simulink model "mfordmodel_v1"  (R2023a)
settings: Solver=ode45  StartTime=0.0  StopTime=10.0  RelTol=1e-3  EnableMultiTasking=on
undefined symbols (not defined in the file): ABV_RATIO_SW, AC_OFF_DLY, ACLOD, AUTO_TRNS_SW, BRAKE_DNDT_X, BZZRPM, BZZRPM_ALT, BZZTM, BZZTM_ALT, CMD_LITOFF, CMD_STABLE, CO_ST_ECT__A, COOL_BASE, DAS_BKDLY_A, DAS_CNT, DAS_CTDLY, DAS_LC_SW__A, DASCLP_5INH, DASCTL, DASMHYST, DASMPH, DEBYCP, DES_BASE, DPNEU_MUL, DSDRPM_DN_TC, DSDRPM_OFF, DSDRPM_UP_TC, EDF_DELAY, EDFHP, ETC_CL_TP, ETC_HP, GR_CM_CREEP, HCAM_ACT_CLP, HEDFHP, HEDFRPM, HICAM_PS, IAC_CAL_SW, IAC_ER_TM1, IAC_ER_TM2, IAC_ER_TM4, IAC_HI_LIM__A, IAC_ISFL_OBD, IAC_KAM_SW, IAC_LO_LIM__A, IAC_MON_TM, IAC_OT_REQ, IAC_RUN_TM, IAC_TP_OBD, IAC_TR_DAS, IAC_TST_DC, ID_DAS__A, ID_NOVS__A, IDVS_CH__A, IDVS_SL__A, IPSI_SW, IPSIDLY, IS_DRBASE__A, IS_DRBASE_A__A, IS_NUBASE__A, IS_NUBASE_A__A ... (+35)
libraries: simulink x2
(part 2 of 12)

== system mfordmodel_v1/iac_v04_001_001/activate_desired_rpm/base_rpm_and_select_logic ==
  note: Note: Be sure to enable C bit-like
      | operations for this chart during test.
  trig_base_rpm_and_select_logic : Inport
  iac_inf_amb : Inport  Port=2
  is_tot_rpm : Inport  Port=3
  is_xtend_rpm : Inport  Port=4
  is_ps_rpm : Inport  Port=5
  is_ac_rpm : Inport  Port=6
  is_alt_rpm : Inport  Port=7
  is_tsl_rpm : Inport  Port=8
  is_hedf_rpm : Inport  Port=9
  er_rpm : Inport  Port=10
  hicam : Inport  Port=11
  dndsup : Inport  Port=12
  alt_cal_flg : Inport  Port=13
  cool_flg : Inport  Port=14
  runup_flg : Inport  Port=15
  iac_dlt_time : Inport  Port=16
  er_isc_req : Inport  Port=17
  base_rpm_and_select_logic_ctl : Stateflow chart  TreatAsAtomicUnit=on
  dsdrpm_calc : Subsystem  TreatAsAtomicUnit=on  mask(do_dsdrpm_calc){}
      mask help: TBD
      mask Display:
      | disp('
      | dsdrpm_lst = dsdrpm;           \n
      | dsdrpm = rolav_tc ( dsdrpm, \n
      |  dsdrpm_tmp,      \n
      |  iac_dlt_time,    \n
      | dsdrpm_tc_tmp)\n
      | ')
  htr_core_rpm_calc : Subsystem  TreatAsAtomicUnit=on  mask(do_htr_core_rpm_calc){}
      mask help: TBD
      mask Display:
      | disp('
      | IF ( ml_heater_core_calc_sw == 1)  THEN        \n
      | is_heater_core_rpm_tmp =               \n
      | fox( FN_NUBASE_IA, iac_inf_amb)\n
      | ELSE IF (ml_heater_core_calc_sw == 2) THEN   \n
      | is_heater_core_rpm_tmp =                \n
      | fox( FN_DRBASE_IA, iac_inf_amb)\n
      | ENDIF                                                          ')
  dsdrpm : Outport
  dsdrpm_lst : Outport  Port=2
  is_source : Outport  Port=3
  wires:
  dsdrpm_calc/2(dsdrpm_lst) -> dsdrpm_lst/1, [dsdrpm_lst]
  [dsdrpm_lst] -> base_rpm_and_select_logic_ctl/14(dsdrpm_lst)
  [do_dsdrpm_calc] -> dsdrpm_calc/Trigger
  iac_dlt_time/1 -> dsdrpm_calc/3(iac_dlt_time)
  base_rpm_and_select_logic_ctl/2(dsdrpm_tmp) -> dsdrpm_calc/1(dsdrpm_tmp)  "dsdrpm_tmp"
  base_rpm_and_select_logic_ctl/3(dsdrpm_tc_tmp) -> dsdrpm_calc/2(dsdrpm_tc_tmp)  "dsdrpm_tc_tmp"
  runup_flg/1 -> base_rpm_and_select_logic_ctl/13(runup_flg)
  cool_flg/1 -> base_rpm_and_select_logic_ctl/12(cool_flg)
  alt_cal_flg/1 -> base_rpm_and_select_logic_ctl/11(alt_cal_flg)
  dndsup/1 -> base_rpm_and_select_logic_ctl/10(dndsup)
  hicam/1 -> base_rpm_and_select_logic_ctl/9(hicam)
  er_rpm/1 -> base_rpm_and_select_logic_ctl/8(er_rpm)
  is_hedf_rpm/1 -> base_rpm_and_select_logic_ctl/7(is_hedf_rpm)
  is_tsl_rpm/1 -> base_rpm_and_select_logic_ctl/6(is_tsl_rpm)
  is_alt_rpm/1 -> base_rpm_and_select_logic_ctl/5(is_alt_rpm)
  is_ac_rpm/1 -> base_rpm_and_select_logic_ctl/4(is_ac_rpm)
  is_ps_rpm/1 -> base_rpm_and_select_logic_ctl/3(is_ps_rpm)
  is_xtend_rpm/1 -> base_rpm_and_select_logic_ctl/2(is_xtend_rpm)
  is_tot_rpm/1 -> base_rpm_and_select_logic_ctl/1(is_tot_rpm)
  htr_core_rpm_calc/1(is_heater_core_rpm_tmp) -> base_rpm_and_select_logic_ctl/16(is_heater_core_rpm_tmp)
  base_rpm_and_select_logic_ctl/4(ml_htr_core_calc_sw) -> htr_core_rpm_calc/1(ml_heater_core_calc_sw)  "ml_heater_core_calc_sw"
  iac_inf_amb/1 -> htr_core_rpm_calc/2(iac_inf_amb)
  base_rpm_and_select_logic_ctl/6(do_htr_core_rpm_calc()) -> htr_core_rpm_calc/Trigger  "do_htr_core_rpm_calc"
  base_rpm_and_select_logic_ctl/1(is_source) -> is_source/1  "is_source"
  base_rpm_and_select_logic_ctl/5(do_dsdrpm_calc()) -> [do_dsdrpm_calc]  "do_dsdrpm_calc"
  trig_base_rpm_and_select_logic/1 -> base_rpm_and_select_logic_ctl/Trigger
  er_isc_req/1 -> base_rpm_and_select_logic_ctl/15(er_isc_req)
  dsdrpm_calc/1(dsdrpm) -> dsdrpm/1

== system mfordmodel_v1/iac_v04_001_001/activate_desired_rpm/hicam_rpm_request ==
  note: Note: Be sure to enable C bit-like
      | operations for this chart during test.
  trig_hicam_rpm_request : Inport
  act : Inport  Port=2
  ect : Inport  Port=3
  acstrt : Inport  Port=4
  tcstrt : Inport  Port=5
  atmr1 : Inport  Port=6
  apt : Inport  Port=7
  crkflg : Inport  Port=8
  ndsflg : Inport  Port=9
  dndsup : Inport  Port=10
  ext_cmd : Inport  Port=11
  alt_cal_flg : Inport  Port=12
  iac_dlt_time : Inport  Port=13
  runup_flg : Inport  Port=14
  fox_calcs : Subsystem  TreatAsAtomicUnit=on  mask(fox_calcs){}
      mask help: TBD
      mask Display:
      | disp('\n
      | ml_fn825b = FN825b(act)               \n
      | ml_fn826b = FN826B(act)               \n
      | ml_fn803a = FN803A(acstrt            \n
      | ml_fn826a = FN826A(tcstrt)            \n
      | ml_fn825a = FN825A(ect)               \n
      | ml_fn825a_alt = FN825A_ALT(ect)\n\n
      | ml_isadd_min = MIN( ml_fn825b,   \n
      | HCAM_ACT_CLP) ')
  hicam_calc : Subsystem  TreatAsAtomicUnit=on  mask(hicam_calc){}
      mask help: TBD
      mask Display:
      | disp('\n
      | IF (ml_isadd_sw == 1) THEN           \n
      |   isadd_ext__A = IS_CMD_ADD \n
      | ELSE IF (ml_isadd_sw == 2) THEN \n
      |   isadd_ext__A = ml_isadd_ext \n
      | ELSE IF (ml_isadd_sw == 3) THEN \n
      |   isadd_ext__A = 0.0                  \n
      | ENDIF                                             \n\n
      | hicam =   isadd_act_tmp                \n
      |                + isadd_ect_tmp     \n
      |                + isadd_st_ect_tmp \n
      |                + isadd_st_act_tmp \n
      |                + isadd_buzz_tmp   \n
      |                + isadd_ext__A        ')
  hicam_rpm_request_ctl : Stateflow chart  TreatAsAtomicUnit=on
  isadd_ramp : Subsystem  TreatAsAtomicUnit=on  mask(isadd_ramp){}
      mask help: If the CAT is cold and the engine is running then ramp the CAT mid rpm adder up. If the CAT is warm (out of deadban) then ramp the rpm adder towards zero because no rpm adder is needed.
      mask Display:
      | disp('\n
      | IF (ml_ramp_sw == 1) THEN               \n
      |  ramp ml_isadd_ext towards          \n
      |  IS_CMD_ADD  with TC = 60 sec. \n
      | ELSE (ml_ramp_sw == 2) THEN         \n
      |   ramp ml_isadd_ext towards         \n
      |   0.0  with TC = 30 sec.                 \n
      | ENDIF                                                 \n
      | ')
  hicam : Outport
  ctptfg : Outport  Port=2
  ptctfg : Outport  Port=3
  wires:
  ext_cmd/1 -> hicam_rpm_request_ctl/7(ext_cmd)
  dndsup/1 -> hicam_rpm_request_ctl/6(dndsup)
  hicam_rpm_request_ctl/9(ptctfg) -> ptctfg/1  "ptctfg"
  hicam_rpm_request_ctl/8(ctptfg) -> ctptfg/1  "ctptfg"
  ndsflg/1 -> hicam_rpm_request_ctl/5(ndsflg)
  crkflg/1 -> hicam_rpm_request_ctl/4(crkflg)
  apt/1 -> hicam_rpm_request_ctl/3(apt)
  atmr1/1 -> hicam_rpm_request_ctl/2(atmr1)
  alt_cal_flg/1 -> hicam_rpm_request_ctl/1(alt_cal_flg)
  fox_calcs/6(ml_fn825a_alt) -> hicam_rpm_request_ctl/10(ml_fn825a_alt)
  fox_calcs/5(ml_fn825a) -> hicam_rpm_request_ctl/11(ml_fn825a)
  fox_calcs/4(ml_fn826b) -> hicam_rpm_request_ctl/12(ml_fn826b)
  fox_calcs/3(ml_fn826a) -> hicam_rpm_request_ctl/13(ml_fn826a)
  fox_calcs/2(ml_fn803a) -> hicam_rpm_request_ctl/14(ml_fn803a)
  fox_calcs/1(ml_fn825b) -> hicam_rpm_request_ctl/15(ml_fn825b)
  hicam_rpm_request_ctl/10(do_hicam_calc()) -> [do_hicam_calc]  "do_hicam_calc"
  trig_hicam_rpm_request/1 -> hicam_rpm_request_ctl/Trigger
  hicam_rpm_request_ctl/12(do_fox_calcs()) -> fox_calcs/Trigger  "do_fox_calcs"
  hicam_rpm_request_ctl/5(isadd_buzz_tmp) -> hicam_calc/5(isadd_buzz_tmp)  "isadd_buzz_tmp"
  hicam_rpm_request_ctl/4(isadd_st_act_tmp) -> hicam_calc/4(isadd_st_act_tmp)  "isadd_st_act_tmp"
  hicam_rpm_request_ctl/3(isadd_st_ect_tmp) -> hicam_calc/3(isadd_st_ect_tmp)  "isadd_st_ect_tmp"
  hicam_rpm_request_ctl/2(isadd_ect_tmp) -> hicam_calc/2(isadd_ect_tmp)  "isadd_ect_tmp"
  hicam_rpm_request_ctl/1(isadd_act_tmp) -> hicam_calc/1(isadd_act_tmp)  "isadd_act_tmp"
  [do_hicam_calc] -> hicam_calc/Trigger
  fox_calcs/7(ml_isadd_min) -> hicam_rpm_request_ctl/9(ml_isadd_min)
  hicam_rpm_request_ctl/6(ml_isadd_sw) -> hicam_calc/6(ml_isadd_sw)  "ml_isadd_sw"
  hicam_rpm_request_ctl/11(do_isadd_ramp()) -> [do_isadd_ramp]  "do_isadd_ramp"
  isadd_ramp/1(ml_isadd_ext) -> hicam_calc/7(ml_isadd_ext)
  hicam_rpm_request_ctl/7(ml_ramp_sw) -> [ml_ramp_sw]  "ml_ramp_sw"
  tcstrt/1 -> fox_calcs/3(tcstrt)
  act/1 -> fox_calcs/1(act)
  runup_flg/1 -> hicam_rpm_request_ctl/8(runup_flg)
  [do_isadd_ramp] -> isadd_ramp/Trigger
  [isadd_ext__A] -> isadd_ramp/2(isadd_ext__A)
  [ml_ramp_sw] -> isadd_ramp/1(ml_ramp_sw)
  iac_dlt_time/1 -> isadd_ramp/3(iac_dlt_time)
  ect/1 -> fox_calcs/4(ect)
  acstrt/1 -> fox_calcs/2(acstrt)
  hicam_calc/1(hicam) -> hicam/1
  hicam_calc/2(isadd_ext__A) -> [isadd_ext__A]

== system mfordmodel_v1/iac_v04_001_001/activate_desired_rpm/inf_amb_calc ==
  ml_inf_amb_sw : Inport
  infamb_kam : Inport  Port=2
  iac_dlt_time : Inport  Port=3
  do_inf_amb_calc : TriggerPort  TriggerType=function-call  VariantControl=(inherit)
  Constant : Constant  Value=254.0
  Multiport Switch : MultiPortSwitch  Inputs=2
  ROLAV_TC_DT_in : Subsystem  mask(Rolling Average - Time Constant){TAU=16}
      mask prompts: TAU "Time Constant"
      mask help: Rolling Average - Time Constant. This filter block is the first order approximation using a time constant. Inputs include the time constant (entered through this dialogue), old_ave which is the previous average value, new_value which is the new filter to filter toward, and the delta_time which is elapsed time over which to perform the filter equation.
      mask init:
      | if isletter(TAU(1))
      |   tc = evalin('base',TAU);
      |   name = TAU;
      | else
      |   tc = str2num(TAU);
      |   name = 'TC';
      | end;
      mask Display: fprintf('%s = %.4f',name,tc);
  Unit Delay : UnitDelay  SampleTime=-1
  iac_inf_amb : Outport
  wires:
  Multiport Switch/1 -> iac_inf_amb/1, Unit Delay/1  "iac_inf_amb"
  ml_inf_amb_sw/1 -> Multiport Switch/1
  infamb_kam/1 -> Multiport Switch/2
  ROLAV_TC_DT_in/1(new_ave) -> Multiport Switch/3  "iac_inf_amb"
  iac_dlt_time/1 -> ROLAV_TC_DT_in/3(delta_time)
  Constant/1 -> ROLAV_TC_DT_in/1(new_value)
  Unit Delay/1 -> ROLAV_TC_DT_in/2(old_ave)

== system mfordmodel_v1/iac_v04_001_001/activate_desired_rpm/rpm_adders_fans_and_pw_steer ==
  trig_rpm_adders_fans_pw_steer : Inport
  hsf_flg : Inport  Port=2
  powsfg : Inport  Port=3
  rpm_adders_fans_pw_steer_ctl : Stateflow chart  TreatAsAtomicUnit=on
  is_hedf_rpm : Outport
  is_ps_rpm : Outport  Port=2
  wires:
  powsfg/1 -> rpm_adders_fans_pw_steer_ctl/2(powsfg)
  hsf_flg/1 -> rpm_adders_fans_pw_steer_ctl/1(hsf_flg)
  rpm_adders_fans_pw_steer_ctl/1(is_hedf_rpm) -> is_hedf_rpm/1  "is_hedf_rpm"
  rpm_adders_fans_pw_steer_ctl/2(is_ps_rpm) -> is_ps_rpm/1  "is_ps_rpm"
  trig_rpm_adders_fans_pw_steer/1 -> rpm_adders_fans_pw_steer_ctl/Trigger

== system mfordmodel_v1/iac_v04_001_001/activate_desired_rpm/rpm_calcs ==
  nobart : Inport
  stb_lold_tmr : Inport  Port=2
  tot : Inport  Port=3
  iac_inf_amb : Inport  Port=4
  ml_tsl_sw : Inport  Port=5
  ml_ac_sw : Inport  Port=6
  ml_xtend_sw : Inport  Port=7
  ml_tot_sw : Inport  Port=8
  do_rpm_calcs : TriggerPort  TriggerType=function-call  VariantControl=(inherit)
  "  4" : Subsystem  mask(Constant){constant=COAST_FRAC}
      mask help: Constant Block. Will dispaly constant name and value on the icon of the block
      mask init:
      | if isletter(constant(1))
      |   const = evalin('base',constant);
      |   name = constant;
      | else
      |   const = str2num(constant);
      |   name = 'CONST';
      | end;
      mask Display: fprintf('%s = %.4f',name,const);
  "  5" : Subsystem  mask(Constant){constant=RT_CHAIN}
      mask help: Constant Block. Will dispaly constant name and value on the icon of the block
      mask init:
      | if isletter(constant(1))
      |   const = evalin('base',constant);
      |   name = constant;
      | else
      |   const = str2num(constant);
      |   name = 'CONST';
      | end;
      mask Display: fprintf('%s = %.4f',name,const);
  Constant : Constant  Value=0.0
  Constant1 : Constant  Value=0.0
  Constant2 : Constant  Value=0.0
  Multiport Switch : MultiPortSwitch  Inputs=2
  Multiport Switch1 : MultiPortSwitch
  Multiport Switch2 : MultiPortSwitch  Inputs=2
  Multiport Switch3 : MultiPortSwitch  Inputs=2
  Product : Product  Inputs=3  InputSameDT=on  RndMeth=Zero  SaturateOnIntegerOverflow=on  OutDataTypeStr=Inherit: Same as first input
  lookup_2d : Subsystem  mask(2-D, piece-wise, linear interpolation){CAL_FUNC=FNIAC_AC_N}
      mask prompts: CAL_FUNC "Calibration function name"
      mask help:
      | Performs piece-wise linear interpolation.
      |
      | Output is NOT extrapolated beyond the input range.  If the input value presented to the block lies outside the range specified in the block's parameter, then the value is treated as though it has the value of the nearest value in the range.
      mask init:
      | if isempty(CAL_FUNC) |  isspace(CAL_FUNC)
      |  calfunc.X=[0 5 10];
      |  calfunc.Y=[0 5 10];
      |  min_x=0;
      |  min_y=0;
      |  max_x=10;
      |  max_y=10;
      |  CAL_FUNC='FNxxx';
      | else
      |   calfunc = evalin('base', CAL_FUNC);
      |   min_x = calfunc.X(1);
      |   min_y = calfunc.Y(1);
      |   max_x = calfunc.X(length(calfunc.X));
      |   max_y = calfunc.Y(length(calfunc.Y));
      | end
      mask Help:
      | Enter the name of the calibration function.
      | (e.g. EGM_VA_ECT_MULT)
      mask Display:
      | fprintf('%s',CAL_FUNC);
      | plot(calfunc.X,calfunc.Y,max_x*1.05,max_y*1.05,min_x,min_y);
  lookup_2d1 : Subsystem  mask(2-D, piece-wise, linear interpolation){CAL_FUNC=FNIAC_AC_D}
      mask prompts: CAL_FUNC "Calibration function name"
      mask help:
      | Performs piece-wise linear interpolation.
      |
      | Output is NOT extrapolated beyond the input range.  If the input value presented to the block lies outside the range specified in the block's parameter, then the value is treated as though it has the value of the nearest value in the range.
      mask init: same as mfordmodel_v1/iac_v04_001_001/activate_desired_rpm/rpm_calcs/lookup_2d
      mask Help:
      | Enter the name of the calibration function.
      | (e.g. EGM_VA_ECT_MULT)
      mask Display:
      | fprintf('%s',CAL_FUNC);
      | plot(calfunc.X,calfunc.Y,max_x*1.05,max_y*1.05,min_x,min_y);
  lookup_2d2 : Subsystem  mask(2-D, piece-wise, linear interpolation){CAL_FUNC=FN861R}
      mask prompts: CAL_FUNC "Calibration function name"
      mask help:
      | Performs piece-wise linear interpolation.
      |
      | Output is NOT extrapolated beyond the input range.  If the input value presented to the block lies outside the range specified in the block's parameter, then the value is treated as though it has the value of the nearest value in the range.
      mask init: same as mfordmodel_v1/iac_v04_001_001/activate_desired_rpm/rpm_calcs/lookup_2d
      mask Help:
      | Enter the name of the calibration function.
      | (e.g. EGM_VA_ECT_MULT)
      mask Display:
      | fprintf('%s',CAL_FUNC);
      | plot(calfunc.X,calfunc.Y,max_x*1.05,max_y*1.05,min_x,min_y);
  lookup_2d3 : Subsystem  mask(2-D, piece-wise, linear interpolation){CAL_FUNC=FN861}
      mask prompts: CAL_FUNC "Calibration function name"
      mask help:
      | Performs piece-wise linear interpolation.
      |
      | Output is NOT extrapolated beyond the input range.  If the input value presented to the block lies outside the range specified in the block's parameter, then the value is treated as though it has the value of the nearest value in the range.
      mask init: same as mfordmodel_v1/iac_v04_001_001/activate_desired_rpm/rpm_calcs/lookup_2d
      mask Help:
      | Enter the name of the calibration function.
      | (e.g. EGM_VA_ECT_MULT)
      mask Display:
      | fprintf('%s',CAL_FUNC);
      | plot(calfunc.X,calfunc.Y,max_x*1.05,max_y*1.05,min_x,min_y);
  lookup_2d4 : Subsystem  mask(2-D, piece-wise, linear interpolation){CAL_FUNC=FN880N}
      mask prompts: CAL_FUNC "Calibration function name"
      mask help:
      | Performs piece-wise linear interpolation.
      |
      | Output is NOT extrapolated beyond the input range.  If the input value presented to the block lies outside the range specified in the block's parameter, then the value is treated as though it has the value of the nearest value in the range.
      mask init: same as mfordmodel_v1/iac_v04_001_001/activate_desired_rpm/rpm_calcs/lookup_2d
      mask Help:
      | Enter the name of the calibration function.
      | (e.g. EGM_VA_ECT_MULT)
      mask Display:
      | fprintf('%s',CAL_FUNC);
      | plot(calfunc.X,calfunc.Y,max_x*1.05,max_y*1.05,min_x,min_y);
  is_tsl_rpm : Outport
  is_ac_rpm : Outport  Port=2
  is_tot_rpm : Outport  Port=3
  is_xtend_rpm : Outport  Port=4
  wires:
  "  5"/1(Out) -> Product/2
  Multiport Switch1/1 -> is_ac_rpm/1  "is_ac_rpm"
  Constant1/1 -> Multiport Switch1/4
  lookup_2d/1(Out1) -> Multiport Switch1/2
  lookup_2d1/1(Out1) -> Multiport Switch1/3
  ml_ac_sw/1 -> Multiport Switch1/1
  iac_inf_amb/1 -> lookup_2d/1(In1), lookup_2d1/1(In1)
  "  4"/1(Out) -> Product/3
  nobart/1 -> Product/1
  lookup_2d2/1(Out1) -> Multiport Switch2/2
  lookup_2d3/1(Out1) -> Multiport Switch2/3
  Multiport Switch2/1 -> is_tot_rpm/1  "is_tot_rpm"
  ml_tot_sw/1 -> Multiport Switch2/1
  tot/1 -> lookup_2d2/1(In1), lookup_2d3/1(In1)
  Constant2/1 -> Multiport Switch3/3
  lookup_2d4/1(Out1) -> Multiport Switch3/2
  Multiport Switch3/1 -> is_xtend_rpm/1  "is_xtend_rpm"
  ml_xtend_sw/1 -> Multiport Switch3/1
  stb_lold_tmr/1 -> lookup_2d4/1(In1)
  Product/1 -> Multiport Switch/3
  Constant/1 -> Multiport Switch/2
  Multiport Switch/1 -> is_tsl_rpm/1  "is_tsl_rpm"
  ml_tsl_sw/1 -> Multiport Switch/1

== system mfordmodel_v1/iac_v04_001_001/iac_executive/fault_code_setting ==
  note: NOTE: Enable 'C-like' bit operations
      | when performing UNIT TEST
      | on this chart.
  trig_fault_code_setting : Inport
  abv_percent : Inport  Port=2
  abv_status : Inport  Port=3
  ccm_ena_flg : Inport  Port=4
  iac_dlt_time : Inport  Port=5
  Constant3 : Constant  Value=0.0
  Constant4 : Constant  Value=0
  Constant5 : Constant
  TIMER_DT_in : Subsystem  mask(TIMER){timer_name=iac_er_tmr4, init_value=0, clipped=off, tmin=, tmax=, unit_str=seconds}
      mask prompts: timer_name "Enter Timer Name"; init_value "initial TIMER value (in seconds)"; clipped "Clip timer?"; tmin "Minimum clip"; tmax "Maximum clip"; unit_str "Select timer units"
      mask help: Acts as a timer. Can count up, down, hold, or reset to zero. The required inputs are a timer function call, a reset function call, a reset value, an increment flag, and a decrement flag. Timer initial value, max and min clip values and timer name are selected below.
      mask init:
      | if ( clipped )
      |   if isletter(tmin(1))
      |     timer_min = evalin('base', tmin);
      |     const_min = timer_min;
      |   else
      |     timer_min = tmin;
      |     tmin = 'Min';
      |     const_min = str2num(timer_min);
      |   end
      |   if isletter(tmax(1))
      |     timer_max = evalin('base', tmax);
      |     const_max = timer_max;
      |   else
      |     timer_max = tmax;
      |     tmax = 'Max';
      |     const_max = str2num(timer_max);
      |   end
      | else
      |   timer_min = 0.0;
      |   const_min = 0.0;
      |   tmin = 'Min';
      |   timer_max = inf;
      |   const_max = inf;
      |    tmax = 'Max';
      | end
      | min_text = strcat(tmin,' = ',num2str(timer_min));
      | max_text = strcat(tmax ,' = ' ,num2str(timer_max));
      | if (strcmp(unit_str, 'seconds' ))
      |   unit_mul = 1;
      |   resolution = 0.000001;
      | else
      |   unit_mul = 1000;
      |    resolution = 1;
      | end
      mask Help:
      | <b><font size="+2">Input/Output Ports</font></b><br>
      | <p>
      | <b>Trig_timer:</b><br>
      | Connect a function call input to the 'trig_timer' port.  A function call passed through this port will activate the TIMER tool.  Activation updates the TIMER output.
      | <p>
      | <b>Trig_reset:</b><br>
      | Connect a function call input to the 'trig_reset' port.  A function call passed through this port will activate the TIMER tool.  Activation resets the TIMER output to the value passed to the 'reset_value' port.
      | <p>
      | <b>Reset_value:</b><br>
      | When 'trig_reset' is activated, the TIMER value will be reset to the real value passed to this input.
      | <p>
      | <b>Increment_flag and decrement_flag:</b><br>
      | If 'increment_flag' is 1 and 'decrement_flag' is 0, TIMER counts up.
      | If 'decrement_flag' is 1 and 'increment_flag' is 0, TIMER counts down.
      | If the flags are both 0 or both 1, TIMER holds its current value.
      | <p>
      | <b><font size="+2">Parameter Selection:</font></b>
      | <p>
      | <b>Initial TIMER Value:</b><br>
      | TIMER will begin at specified value.  Enter in seconds.
      mask TypeOptions unit_str: seconds | milliseconds
      mask Display:
      | plot( [0.3 0.45 0.55 0.7], [0.4 0.4 0.6 0.6])
      | plot( [ .475 .435 .415  .4 .4  .415 .435 .475  .525 .565 .585 .6 .6  ...
      | .585 .565 .525 .475], [.9  .885 .865  .825 .775 .735 .715  .7 .7 ...
      | .715 .735 .775 .825  .865 .885 .9 .9] )
      | plot( [.5 .5], [.89 .87])
      | plot( [.5 .5], [.71 .73])
      | plot( [.41 .43], [.8 .8])
      | plot( [.57 .59], [.8 .8])
      | plot( [.5 .5], [.8 .89])
      | plot( [.49 .5 .51], [.88 .89 .88] )
      | plot( [.5 .555], [.8 .825] )
      | plot( [.535 .555 .555], [.825 .825 .815])
      | text(0.35, 0.35, min_text)
      | text(0.6, 0.7,max_text)
      | text( 0.35, .95, timer_name)
  fault_code_setting_ctl : Stateflow chart  TreatAsAtomicUnit=on
  type1_fault_code : Subsystem  mask(fault code){pcode=1504, ms=CCM}
      mask prompts: pcode "Code Number (e.g. 1234)"; ms "System ID"
      mask help: Gereric Fault Code - NOT functional
      mask init:
      | if (pcode == 'xxxx')
      | pcode_num = 0;
      | else
      | pcode_num = str2num(pcode);
      | end
      | mon_select=eval('ms');
      mask TypeOptions ms: CCM | CAT | PURG | SAIR | EGR | EGO | COOL | FCAP | P0456
      mask Display: fprintf('P%s\n%s',pcode,ms);
  p1504 : Outport
  wires:
  type1_fault_code/1(pxxxx) -> p1504/1  "p1504"
  Constant5/1 -> TIMER_DT_in/4(inc flag)
  Constant4/1 -> TIMER_DT_in/5(dec flag)
  Constant3/1 -> TIMER_DT_in/3(reset value)
  iac_dlt_time/1 -> TIMER_DT_in/6(delta time)
  fault_code_setting_ctl/1(trig_incr_tmr4()) -> TIMER_DT_in/1(trig_time)  "trig_incr_tmr4"
  fault_code_setting_ctl/2(trig_rst_tmr4()) -> TIMER_DT_in/2(trig_reset)  "trig_rst_tmr4"
  TIMER_DT_in/1(timer) -> fault_code_setting_ctl/4(iac_er_tmr4)  "iac_er_tmr4"
  trig_fault_code_setting/1 -> fault_code_setting_ctl/Trigger
  fault_code_setting_ctl/3(trig_set_p1504_malf()) -> type1_fault_code/1(trig_malfunction)  "trig_set_p1504_malf"
  fault_code_setting_ctl/4(trig_clear_p1504_malf()) -> type1_fault_code/2(trig_clear_malf)  "trig_clear_p1504_malf"
  ccm_ena_flg/1 -> fault_code_setting_ctl/3(ccm_ena_flg)
  abv_status/1 -> fault_code_setting_ctl/2(abv_status)
  abv_percent/1 -> fault_code_setting_ctl/1(abv_percent)

== system mfordmodel_v1/iac_v04_001_001/iac_executive/iac_dlt_time_calc ==
  do_iac_dlt_time_calc : TriggerPort  TriggerType=function-call  VariantControl=(inherit)
  Digital Clock : DigitalClock  SampleTime=-1
  Sum : Sum  Inputs=+-  InputSameDT=on  SaturateOnIntegerOverflow=on  OutDataTypeStr=Inherit: Same as first input
  Unit Delay : UnitDelay  SampleTime=-1
  iac_dlt_time : Outport  InitialOutput=0
  wires:
  Digital Clock/1 -> Unit Delay/1, Sum/1
  Sum/1 -> iac_dlt_time/1  "iac_dlt_time"
  Unit Delay/1 -> Sum/2

== system mfordmodel_v1/iac_v04_001_001/iac_executive/misc_calcs ==
  trig_misc_calcs : Inport
  dndti : Inport  Port=2
  iac_dlt_time : Inport  Port=3
  subst_req_0 : Inport  Port=4
  tslpip : Inport  Port=5
  runup_flg : Inport  Port=6
  crkflg : Inport  Port=7
  er_isc_hld : Inport  Port=8
  mfmflg : Inport  Port=9
  tfmflg : Inport  Port=10
  eng_stalled : Inport  Port=11
  gr_cm : Inport  Port=12
  apt : Inport  Port=13
  Constant3 : Constant  Value=0.0
  Constant4 : Constant  Value=0
  Constant5 : Constant
  TIMER_DT_in : Subsystem  mask(TIMER){timer_name=gear5tmr, init_value=0, clipped=on, tmin=0, tmax=31.75, unit_str=seconds}
      mask prompts: timer_name "Enter Timer Name"; init_value "initial TIMER value (in seconds)"; clipped "Clip timer?"; tmin "Minimum clip"; tmax "Maximum clip"; unit_str "Select timer units"
      mask help: Acts as a timer. Can count up, down, hold, or reset to zero. The required inputs are a timer function call, a reset function call, a reset value, an increment flag, and a decrement flag. Timer initial value, max and min clip values and timer name are selected below.
      mask init: same as mfordmodel_v1/iac_v04_001_001/iac_executive/fault_code_setting/TIMER_DT_in
      mask Help:
      | <b><font size="+2">Input/Output Ports</font></b><br>
      | <p>
      | <b>Trig_timer:</b><br>
      | Connect a function call input to the 'trig_timer' port.  A function call passed through this port will activate the TIMER tool.  Activation updates the TIMER output.
      | <p>
      | <b>Trig_reset:</b><br>
      | Connect a function call input to the 'trig_reset' port.  A function call passed through this port will activate the TIMER tool.  Activation resets the TIMER output to the value passed to the 'reset_value' port.
      | <p>
      | <b>Reset_value:</b><br>
      | When 'trig_reset' is activated, the TIMER value will be reset to the real value passed to this input.
      | <p>
      | <b>Increment_flag and decrement_flag:</b><br>
      | If 'increment_flag' is 1 and 'decrement_flag' is 0, TIMER counts up.
      | If 'decrement_flag' is 1 and 'increment_flag' is 0, TIMER counts down.
      | If the flags are both 0 or both 1, TIMER holds its current value.
      | <p>
      | <b><font size="+2">Parameter Selection:</font></b>
      | <p>
      | <b>Initial TIMER Value:</b><br>
      | TIMER will begin at specified value.  Enter in seconds.
      mask TypeOptions unit_str: seconds | milliseconds
      mask Display:
      | plot( [0.3 0.45 0.55 0.7], [0.4 0.4 0.6 0.6])
      | plot( [ .475 .435 .415  .4 .4  .415 .435 .475  .525 .565 .585 .6 .6  ...
      | .585 .565 .525 .475], [.9  .885 .865  .825 .775 .735 .715  .7 .7 ...
      | .715 .735 .775 .825  .865 .885 .9 .9] )
      | plot( [.5 .5], [.89 .87])
      | plot( [.5 .5], [.71 .73])
      | plot( [.41 .43], [.8 .8])
      | plot( [.57 .59], [.8 .8])
      | plot( [.5 .5], [.8 .89])
      | plot( [.49 .5 .51], [.88 .89 .88] )
      | plot( [.5 .555], [.8 .825] )
      | plot( [.535 .555 .555], [.825 .825 .815])
      | text(0.35, 0.35, min_text)
      | text(0.6, 0.7,max_text)
      | text( 0.35, .95, timer_name)
  dndt_calc : Subsystem  TreatAsAtomicUnit=on  mask(dndt_calc){}
      mask help: Filter the rate of change of RPM for use in DASPOT calculations.
      mask Display:
      | disp('\n
      | IF (ml_dndt_sw == 1) THEN          \n
      | dndt_das = 0.0                       \n
      | ELSE IF (ml_dndt_sw == 2) THEN\n
      | dndt_das =  rolav( dndt_das,  \n
      | dndti, iac_dlt_time,\n
      | TCNDT_DAS)          \n
      | ENDIF                                            ')
  misc_calcs_ctl : Stateflow chart  TreatAsAtomicUnit=on
  osc_response_logic_ctl : Stateflow chart  TreatAsAtomicUnit=on
  osc_response_triggered : Subsystem  TreatAsAtomicUnit=on  mask(substitute){resp=22, channel=0}
      mask prompts: resp "Enter Response Code in HEX"; channel "Select OSC channel"
      mask help:
      | This block will perform Output State Control Response, for now it is stub block.
      | Enter the response code and OSC channel number below.
      mask TypeOptions channel: 0 | 1 | 2 | 3 | 4 | 5 | 6 | 7 | 8 | 9 | 10 | 11 | 12 | 15 | 16 | 17 | 18 | 19 | 20 | 21 | 22 | 23 | 24 | 25 | 26 | 27 | 28 | 29 | 30 | 31 | 32 | 33 | 34 | 35 | 36 | 37 | 38 | 39 | 40 | 41 | 42 | 43 | 44 | 45 | 46 | 47 | 48 | 49 | 50
      mask Display: fprintf('\nChannel # = %s\nResponse Code = 0x%s\n',channel,resp);
  gear5tmr : Outport
  gear5th : Outport  Port=2
  dndt_das : Outport  Port=3
  wires:
  apt/1 -> misc_calcs_ctl/3(apt)
  gr_cm/1 -> misc_calcs_ctl/2(gr_cm)
  eng_stalled/1 -> misc_calcs_ctl/1(eng_stalled)
  tslpip/1 -> osc_response_logic_ctl/7(tslpip)
  tfmflg/1 -> osc_response_logic_ctl/6(tfmflg)
  subst_req_0/1 -> osc_response_logic_ctl/5(subst_req_0)
  mfmflg/1 -> osc_response_logic_ctl/4(mfmflg)
  er_isc_hld/1 -> osc_response_logic_ctl/3(er_isc_hld)
  crkflg/1 -> osc_response_logic_ctl/2(crkflg)
  runup_flg/1 -> osc_response_logic_ctl/1(runup_flg)
  misc_calcs_ctl/6(trig_osc_response_logic()) -> osc_response_logic_ctl/Trigger  "trig_osc_response_logic"
  osc_response_logic_ctl/1(do_osc_response()) -> osc_response_triggered/Trigger  "do_osc_responnse"
  dndti/1 -> dndt_calc/2(dndti)
  [ml_dndt_sw] -> dndt_calc/1(ml_dndt_sw)
  misc_calcs_ctl/2(ml_dndt_sw) -> [ml_dndt_sw]  "ml_dndt_sw"
  dndt_calc/1(dndt_das) -> dndt_das/1
  iac_dlt_time/1 -> dndt_calc/3(iac_dlt_time), TIMER_DT_in/6(delta time)
  misc_calcs_ctl/5(do_dndt_calc()) -> dndt_calc/Trigger  "do_dndt_calc"
  Constant3/1 -> TIMER_DT_in/3(reset value)
  Constant4/1 -> TIMER_DT_in/5(dec flag)
  Constant5/1 -> TIMER_DT_in/4(inc flag)
  misc_calcs_ctl/1(gear5th) -> gear5th/1  "gear5th"
  TIMER_DT_in/1(timer) -> gear5tmr/1  "gear5tmr"
  trig_misc_calcs/1 -> misc_calcs_ctl/Trigger
  misc_calcs_ctl/4(trig_rst_gear5tmr()) -> TIMER_DT_in/2(trig_reset)  "trig_rst_gear5tmr"
  misc_calcs_ctl/3(trig_incr_gear5tmr()) -> TIMER_DT_in/1(trig_time)  "trig_incr_gear5tmr"

== system mfordmodel_v1/iac_v04_001_001/iac_executive/mode_control ==
  trig_external_override_mode : Inport
  trig_crank_mode : Inport  Port=2
  do_failure_mode : Inport  Port=3
  osm_eo_off : Inport  Port=4
  osm_eo_on : Inport  Port=5
  osc_ena_0 : Inport  Port=6
  osc_state : Inport  Port=7
  tcstrt : Inport  Port=8
  tslpip : Inport  Port=9
  abv_flowrate_in : Inport  Port=10
  ratch : Inport  Port=11
  abv_ratio_in : Inport  Port=12
  Mux3 : Mux  Inputs=3
  Mux4 : Mux  Inputs=3
  Mux5 : Mux  Inputs=2
  Mux6 : Mux  Inputs=2
  crank_mode : Subsystem
  external_override_mode : Subsystem
  failure_mode : Subsystem  TreatAsAtomicUnit=on  mask(failure_mode){}
      mask help: TBD
      mask Display:
      | disp('abv_flowrate = IAC_FM_PPM\n
      | abv_ratio = 0\n
      | hcamfg = 1\n
      | iscflg = 0')
  abv_flowrate : Outport
  abv_ratio : Outport  Port=2
  hcamfg : Outport  Port=3
  iscflg : Outport  Port=4
  dstpbr : Outport  Port=5
  wires:
  failure_mode/3(hcamfg) -> Mux5/2
  crank_mode/4(iscflg) -> Mux6/1
  failure_mode/4(iscflg) -> Mux6/2
  Mux6/1 -> iscflg/1
  crank_mode/3(hcamfg) -> Mux5/1
  Mux5/1 -> hcamfg/1
  ratch/1 -> crank_mode/4(ratch)
  crank_mode/5(dstpbr) -> dstpbr/1
  crank_mode/1(abv_flowrate) -> Mux3/2
  tslpip/1 -> crank_mode/3(tslpip)
  tcstrt/1 -> crank_mode/2(tcstrt)
  trig_crank_mode/1 -> crank_mode/1(trig_crank_mode)
  crank_mode/2(abv_ratio) -> Mux4/2
  failure_mode/1(abv_flowrate) -> Mux3/3
  do_failure_mode/1 -> failure_mode/Trigger
  failure_mode/2(abv_ratio) -> Mux4/3
  abv_ratio_in/1 -> external_override_mode/7(abv_ratio_in)
  Mux3/1 -> abv_flowrate/1
  Mux4/1 -> abv_ratio/1
  external_override_mode/1(abv_flowrate) -> Mux3/1
  abv_flowrate_in/1 -> external_override_mode/6(abv_flowrate_in)
  external_override_mode/2(abv_ratio) -> Mux4/1
  osc_state/1 -> external_override_mode/5(osc_state)
  osc_ena_0/1 -> external_override_mode/4(osc_ena_0)
  osm_eo_on/1 -> external_override_mode/3(osm_eo_on)
  osm_eo_off/1 -> external_override_mode/2(osm_eo_off)
  trig_external_override_mode/1 -> external_override_mode/1(trig_external_override_mode)

== system mfordmodel_v1/iac_v04_001_001/iac_executive/runup_flag_timer ==
  trig_runup_flag_timer : Inport
  dsdrpm : Inport  Port=2
  alt_cal_flg : Inport  Port=3
  eng_stalled : Inport  Port=4
  engine_speed : Inport  Port=5
  iac_dlt_time : Inport  Port=6
  Constant : Constant  Value=0.0
  Constant1 : Constant
  Constant2 : Constant  Value=0
  TIMER_DT_in : Subsystem  mask(TIMER){timer_name=runuptmr, init_value=0, clipped=off, tmin=, tmax=, unit_str=seconds}
      mask prompts: timer_name "Enter Timer Name"; init_value "initial TIMER value (in seconds)"; clipped "Clip timer?"; tmin "Minimum clip"; tmax "Maximum clip"; unit_str "Select timer units"
      mask help: Acts as a timer. Can count up, down, hold, or reset to zero. The required inputs are a timer function call, a reset function call, a reset value, an increment flag, and a decrement flag. Timer initial value, max and min clip values and timer name are selected below.
      mask init: same as mfordmodel_v1/iac_v04_001_001/iac_executive/fault_code_setting/TIMER_DT_in
      mask Help:
      | <b><font size="+2">Input/Output Ports</font></b><br>
      | <p>
      | <b>Trig_timer:</b><br>
      | Connect a function call input to the 'trig_timer' port.  A function call passed through this port will activate the TIMER tool.  Activation updates the TIMER output.
      | <p>
      | <b>Trig_reset:</b><br>
      | Connect a function call input to the 'trig_reset' port.  A function call passed through this port will activate the TIMER tool.  Activation resets the TIMER output to the value passed to the 'reset_value' port.
      | <p>
      | <b>Reset_value:</b><br>
      | When 'trig_reset' is activated, the TIMER value will be reset to the real value passed to this input.
      | <p>
      | <b>Increment_flag and decrement_flag:</b><br>
      | If 'increment_flag' is 1 and 'decrement_flag' is 0, TIMER counts up.
      | If 'decrement_flag' is 1 and 'increment_flag' is 0, TIMER counts down.
      | If the flags are both 0 or both 1, TIMER holds its current value.
      | <p>
      | <b><font size="+2">Parameter Selection:</font></b>
      | <p>
      | <b>Initial TIMER Value:</b><br>
      | TIMER will begin at specified value.  Enter in seconds.
      mask TypeOptions unit_str: seconds | milliseconds
      mask Display:
      | plot( [0.3 0.45 0.55 0.7], [0.4 0.4 0.6 0.6])
      | plot( [ .475 .435 .415  .4 .4  .415 .435 .475  .525 .565 .585 .6 .6  ...
      | .585 .565 .525 .475], [.9  .885 .865  .825 .775 .735 .715  .7 .7 ...
      | .715 .735 .775 .825  .865 .885 .9 .9] )
      | plot( [.5 .5], [.89 .87])
      | plot( [.5 .5], [.71 .73])
      | plot( [.41 .43], [.8 .8])
      | plot( [.57 .59], [.8 .8])
      | plot( [.5 .5], [.8 .89])
      | plot( [.49 .5 .51], [.88 .89 .88] )
      | plot( [.5 .555], [.8 .825] )
      | plot( [.535 .555 .555], [.825 .825 .815])
      | text(0.35, 0.35, min_text)
      | text(0.6, 0.7,max_text)
      | text( 0.35, .95, timer_name)
  runup_flag_timer_ctl : Stateflow chart  TreatAsAtomicUnit=on
  runup_flg : Outport
  runuptmr : Outport  Port=2
  wires:
  iac_dlt_time/1 -> TIMER_DT_in/6(delta time)
  Constant2/1 -> TIMER_DT_in/5(dec flag)
  Constant1/1 -> TIMER_DT_in/4(inc flag)
  Constant/1 -> TIMER_DT_in/3(reset value)
  TIMER_DT_in/1(timer) -> runuptmr/1  "runuptmr"
  trig_runup_flag_timer/1 -> runup_flag_timer_ctl/Trigger
  runup_flag_timer_ctl/3(trig_rst_runup_tmr()) -> TIMER_DT_in/2(trig_reset)  "trig_rst_runup_tmr"
  runup_flag_timer_ctl/2(trig_incr_runup_tmr()) -> TIMER_DT_in/1(trig_time)  "trig_incr_runup_tmr"
  runup_flag_timer_ctl/1(runup_flg) -> runup_flg/1  "runup_flg"
  dsdrpm/1 -> runup_flag_timer_ctl/1(dsdrpm)
  engine_speed/1 -> runup_flag_timer_ctl/4(engine_speed)
  eng_stalled/1 -> runup_flag_timer_ctl/3(eng_stalled)
  alt_cal_flg/1 -> runup_flag_timer_ctl/2(alt_cal_flg)

== system mfordmodel_v1/iac_v04_001_001/normal_mode/activate_feedforward ==
  trig_activate_feedforward : Inport
  iac_inf_amb : Inport  Port=2
  dsdrpm : Inport  Port=3
  idle_ppm : Inport  Port=4
  hicam : Inport  Port=5
  iac_dlt_time : Inport  Port=6
  atmr3 : Inport  Port=7
  apt : Inport  Port=8
  cool_flg : Inport  Port=9
  ect : Inport  Port=10
  vspd : Inport  Port=11
  engine_speed : Inport  Port=12
  tot : Inport  Port=13
  pdl : Inport  Port=14
  gr_cm : Inport  Port=15
  dndsup : Inport  Port=16
  alt_ppm : Inport  Port=17
  ac_cycle_flg : Inport  Port=18
  ac_ppm_rqst : Inport  Port=19
  powsfg : Inport  Port=20
  vsf : Inport  Port=21
  fantmr : Inport  Port=22
  lsf_rqst : Inport  Port=23
  pstmr : Inport  Port=24
  vfd : Inport  Port=25
  Constant : Constant  Value=0.0
  Constant1 : Constant  Value=0
  Constant2 : Constant
  ac_ppm_tmr : Subsystem  mask(TIMER){timer_name=ac_ppm_tmr, init_value=0, clipped=off, tmin=, tmax=, unit_str=seconds}
      mask prompts: timer_name "Enter Timer Name"; init_value "initial TIMER value (in seconds)"; clipped "Clip timer?"; tmin "Minimum clip"; tmax "Maximum clip"; unit_str "Select timer units"
      mask help: Acts as a timer. Can count up, down, hold, or reset to zero. The required inputs are a timer function call, a reset function call, a reset value, an increment flag, and a decrement flag. Timer initial value, max and min clip values and timer name are selected below.
      mask init:
      | if ( clipped )
      |   if isletter(tmin(1))
      |     timer_min = evalin('base', tmin);
      |     const_min = timer_min;
      |   else
      |     timer_min = tmin;
      |     tmin = 'Min';
      |     const_min = str2num(timer_min);
      |   end
      |   if isletter(tmax(1))
      |     timer_max = evalin('base', tmax);
      |     const_max = timer_max;
      |   else
      |     timer_max = tmax;
      |     tmax = 'Max';
      |     const_max = str2num(timer_max);
      |   end
      | else
      |   timer_min = 0.0;
      |   const_min = 0.0;
      |   tmin = 'Min';
      |   timer_max = inf;
      |   const_max = inf;
      |    tmax = 'Max';
      | end
      | min_text = strcat(tmin,' = ',num2str(timer_min));
      | max_text = strcat(tmax ,' = ' ,num2str(timer_max));
      | if (strcmp(unit_str, 'seconds' ))
      |   unit_mul = 1;
      |   resolution = 0.000001;
      | else
      |   unit_mul = 1000;
      |   resolution = 1;
      | end
      mask Help:
      | <b><font size="+2">Input/Output Ports</font></b><br>
      | <p>
      | <b>Trig_timer:</b><br>
      | Connect a function call input to the 'trig_timer' port.  A function call passed through this port will activate the TIMER tool.  Activation updates the TIMER output.
      | <p>
      | <b>Trig_reset:</b><br>
      | Connect a function call input to the 'trig_reset' port.  A function call passed through this port will activate the TIMER tool.  Activation resets the TIMER output to the value passed to the 'reset_value' port.
      | <p>
      | <b>Reset_value:</b><br>
      | When 'trig_reset' is activated, the TIMER value will be reset to the real value passed to this input.
      | <p>
      | <b>Increment_flag and decrement_flag:</b><br>
      | If 'increment_flag' is 1 and 'decrement_flag' is 0, TIMER counts up.
      | If 'decrement_flag' is 1 and 'increment_flag' is 0, TIMER counts down.
      | If the flags are both 0 or both 1, TIMER holds its current value.
      | <p>
      | <b><font size="+2">Parameter Selection:</font></b>
      | <p>
      | <b>Initial TIMER Value:</b><br>
      | TIMER will begin at specified value.  Enter in seconds.
      mask TypeOptions unit_str: seconds | milliseconds
      mask Display:
      | plot( [0.3 0.45 0.55 0.7], [0.4 0.4 0.6 0.6])
      | plot( [ .475 .435 .415  .4 .4  .415 .435 .475  .525 .565 .585 .6 .6  ...
      | .585 .565 .525 .475], [.9  .885 .865  .825 .775 .735 .715  .7 .7 ...
      | .715 .735 .775 .825  .865 .885 .9 .9] )
      | plot( [.5 .5], [.89 .87])
      | plot( [.5 .5], [.71 .73])
      | plot( [.41 .43], [.8 .8])
      | plot( [.57 .59], [.8 .8])
      | plot( [.5 .5], [.8 .89])
      | plot( [.49 .5 .51], [.88 .89 .88] )
      | plot( [.5 .555], [.8 .825] )
      | plot( [.535 .555 .555], [.825 .825 .815])
      | text(0.35, 0.35, min_text)
      | text(0.6, 0.7,max_text)
      | text( 0.35, .95, timer_name)
  activate_feedforward_ctl : Stateflow chart  TreatAsAtomicUnit=on
  desmaf_pre_calc : Subsystem  TreatAsAtomicUnit=on
  desmaf_pre : Outport
  wires:
  Constant/1 -> ac_ppm_tmr/3(reset value)
  Constant1/1 -> ac_ppm_tmr/5(dec flag)
  Constant2/1 -> ac_ppm_tmr/4(inc flag)
  vfd/1 -> desmaf_pre_calc/18(vfd)
  vsf/1 -> desmaf_pre_calc/17(vsf)
  pstmr/1 -> desmaf_pre_calc/16(pstmr)
  [ect] -> desmaf_pre_calc/7(ect)
  [vspd] -> desmaf_pre_calc/8(vspd)
  dsdrpm/1 -> desmaf_pre_calc/9(dsdrpm)
  tot/1 -> desmaf_pre_calc/11(tot)
  atmr3/1 -> desmaf_pre_calc/10(atmr3)
  engine_speed/1 -> desmaf_pre_calc/12(engine_speed)
  iac_dlt_time/1 -> desmaf_pre_calc/13(iac_dlt_time)
  iac_inf_amb/1 -> desmaf_pre_calc/14(iac_inf_amb)
  alt_ppm/1 -> desmaf_pre_calc/15(alt_ppm)
  ect/1 -> activate_feedforward_ctl/2(ect), [ect]
  dndsup/1 -> activate_feedforward_ctl/1(dndsup)
  vspd/1 -> activate_feedforward_ctl/6(vspd), [vspd]
  desmaf_pre_calc/1(desmaf_pre) -> desmaf_pre/1
  activate_feedforward_ctl/6(ml_fan_sw) -> desmaf_pre_calc/6(ml_fan_sw)  "ml_fan_sw"
  fantmr/1 -> activate_feedforward_ctl/14(fantmr)
  lsf_rqst/1 -> activate_feedforward_ctl/13(lsf_rqst)
  ac_ppm_tmr/1(timer) -> desmaf_pre_calc/19(ac_ppm_tmr)  "ac_ppm_tmr"
  [do_desmaf_pre_calc] -> desmaf_pre_calc/Trigger
  activate_feedforward_ctl/4(ml_base_sw) -> desmaf_pre_calc/4(ml_base_sw)  "ml_base_sw"
  activate_feedforward_ctl/5(ml_trans_sw) -> desmaf_pre_calc/5(ml_trans_sw)  "ml_trans_sw"
  activate_feedforward_ctl/7(do_desmaf_pre_calc()) -> [do_desmaf_pre_calc]  "do_desmaf_pre_calc"
  trig_activate_feedforward/1 -> activate_feedforward_ctl/Trigger
  activate_feedforward_ctl/1(ml_ac_sw) -> desmaf_pre_calc/1(ml_ac_sw)  "ml_ac_sw"
  activate_feedforward_ctl/3(ml_fsc_sw) -> desmaf_pre_calc/3(ml_fsc_sw)  "ml_fsc_sw"
  activate_feedforward_ctl/2(ml_ps_sw) -> desmaf_pre_calc/2(ml_ps_sw)  "ml_ps_sw"
  activate_feedforward_ctl/9(trig_ac_ppm_tmr_reset()) -> ac_ppm_tmr/2(trig_reset)  "trig_ac_ppm_tmr_reset"
  activate_feedforward_ctl/8(trig_ac_ppm_tmr_update()) -> ac_ppm_tmr/1(trig_time)  "trig_ac_ppm_tmr_update"
  hicam/1 -> activate_feedforward_ctl/12(hicam)
  cool_flg/1 -> activate_feedforward_ctl/11(cool_flg)
  powsfg/1 -> activate_feedforward_ctl/10(powsfg)
  ac_cycle_flg/1 -> activate_feedforward_ctl/8(ac_cycle_flg)
  gr_cm/1 -> activate_feedforward_ctl/7(gr_cm)
  apt/1 -> activate_feedforward_ctl/5(apt)
  pdl/1 -> activate_feedforward_ctl/4(pdl)
  idle_ppm/1 -> activate_feedforward_ctl/3(idle_ppm)
  ac_ppm_rqst/1 -> activate_feedforward_ctl/9(ac_ppm_rqst)
